simulink model "model"  (R2014a)
(part 5 of 5)

  L_117853438/LConn3 -- T_117853438__/RConn3 -- bus369/LConn1
  T_140066772__/RConn1 -- L_140066772/LConn1
  T_140066772__/RConn2 -- L_140066772/LConn2
  L_140066772/LConn3 -- T_140066772__/RConn3 -- bus370/LConn1
  T_314931464__Csorna_alállomás/RConn1 -- L_314931464/LConn1
  T_314931464__Csorna_alállomás/RConn2 -- L_314931464/LConn2
  L_314931464/LConn3 -- T_314931464__Csorna_alállomás/RConn3 -- bus371/LConn1
  T_313625037__Pápa_alállomás/RConn1 -- L_313625037/LConn1
  T_313625037__Pápa_alállomás/RConn2 -- L_313625037/LConn2
  L_313625037/LConn3 -- T_313625037__Pápa_alállomás/RConn3 -- bus372/LConn1
  T_370667810__/RConn1 -- L_370667810/LConn1
  T_370667810__/RConn2 -- L_370667810/LConn2
  L_370667810/LConn3 -- T_370667810__/RConn3 -- bus373/LConn1
  T_280595113__/RConn1 -- L_280595113/LConn1
  T_280595113__/RConn2 -- L_280595113/LConn2
  L_280595113/LConn3 -- T_280595113__/RConn3 -- bus374/LConn1
  T_294895233__/RConn1 -- L_294895233/LConn1
  T_294895233__/RConn2 -- L_294895233/LConn2
  L_294895233/LConn3 -- T_294895233__/RConn3 -- bus375/LConn1
  T_253119622__Tamási_alállomás/RConn1 -- L_253119622/LConn1
  T_253119622__Tamási_alállomás/RConn2 -- L_253119622/LConn2
  L_253119622/LConn3 -- T_253119622__Tamási_alállomás/RConn3 -- bus376/LConn1
  T_104062255__Sárbogárd_alállomás/RConn1 -- L_104062255/LConn1
  T_104062255__Sárbogárd_alállomás/RConn2 -- L_104062255/LConn2
  L_104062255/LConn3 -- T_104062255__Sárbogárd_alállomás/RConn3 -- bus377/LConn1
  T_135952041_120000_/RConn1 -- L_135952041/LConn1
  T_135952041_120000_/RConn2 -- L_135952041/LConn2
  L_135952041/LConn3 -- T_135952041_120000_/RConn3 -- bus378/LConn1
  T_350948497__/RConn1 -- L_350948497/LConn1
  T_350948497__/RConn2 -- L_350948497/LConn2
  L_350948497/LConn3 -- T_350948497__/RConn3 -- bus379/LConn1
  T_288254104__/RConn1 -- L_288254104/LConn1
  T_288254104__/RConn2 -- L_288254104/LConn2
  L_288254104/LConn3 -- T_288254104__/RConn3 -- bus380/LConn1
  T_234987164__/RConn1 -- L_234987164/LConn1
  T_234987164__/RConn2 -- L_234987164/LConn2
  L_234987164/LConn3 -- T_234987164__/RConn3 -- bus381/LConn1
  T_110253534__/RConn1 -- L_110253534/LConn1
  T_110253534__/RConn2 -- L_110253534/LConn2
  L_110253534/LConn3 -- T_110253534__/RConn3 -- bus382/LConn1
  T_275352278__Kapuvár_alállomás/RConn1 -- L_275352278/LConn1
  T_275352278__Kapuvár_alállomás/RConn2 -- L_275352278/LConn2
  L_275352278/LConn3 -- T_275352278__Kapuvár_alállomás/RConn3 -- bus383/LConn1
  T_287201135__Békés_120_kV_alállomás/RConn1 -- L_287201135/LConn1
  T_287201135__Békés_120_kV_alállomás/RConn2 -- L_287201135/LConn2
  L_287201135/LConn3 -- T_287201135__Békés_120_kV_alállomás/RConn3 -- bus384/LConn1
  T_302147975__Borsodnádasd_alállomás/RConn1 -- L_302147975/LConn1
  T_302147975__Borsodnádasd_alállomás/RConn2 -- L_302147975/LConn2
  L_302147975/LConn3 -- T_302147975__Borsodnádasd_alállomás/RConn3 -- bus385/LConn1
  T_355349327__Öntödei_alállomás/RConn1 -- L_355349327/LConn1
  T_355349327__Öntödei_alállomás/RConn2 -- L_355349327/LConn2
  L_355349327/LConn3 -- T_355349327__Öntödei_alállomás/RConn3 -- bus386/LConn1
  T_103950678__Dunakeszi_alállomás/RConn1 -- L_103950678/LConn1
  T_103950678__Dunakeszi_alállomás/RConn2 -- L_103950678/LConn2
  L_103950678/LConn3 -- T_103950678__Dunakeszi_alállomás/RConn3 -- bus387/LConn1
  T_103950687_120000_Fót_alállomás/RConn1 -- L_103950687/LConn1
  T_103950687_120000_Fót_alállomás/RConn2 -- L_103950687/LConn2
  L_103950687/LConn3 -- T_103950687_120000_Fót_alállomás/RConn3 -- bus388/LConn1
  T_287114424__/RConn1 -- L_287114424/LConn1
  T_287114424__/RConn2 -- L_287114424/LConn2
  L_287114424/LConn3 -- T_287114424__/RConn3 -- bus389/LConn1
  T_291223737__Kunszentmárton_alállomás/RConn1 -- L_291223737/LConn1
  T_291223737__Kunszentmárton_alállomás/RConn2 -- L_291223737/LConn2
  L_291223737/LConn3 -- T_291223737__Kunszentmárton_alállomás/RConn3 -- bus390/LConn1
  T_288736592__Szentes_alállomás/RConn1 -- L_288736592/LConn1
  T_288736592__Szentes_alállomás/RConn2 -- L_288736592/LConn2
  L_288736592/LConn3 -- T_288736592__Szentes_alállomás/RConn3 -- bus391/LConn1
  T_235409083__Sikonda_alállomás/RConn1 -- L_235409083/LConn1
  T_235409083__Sikonda_alállomás/RConn2 -- L_235409083/LConn2
  L_235409083/LConn3 -- T_235409083__Sikonda_alállomás/RConn3 -- bus392/LConn1
  T_331463129__Mindszentgodisa_alállomás/RConn1 -- L_331463129/LConn1
  T_331463129__Mindszentgodisa_alállomás/RConn2 -- L_331463129/LConn2
  L_331463129/LConn3 -- T_331463129__Mindszentgodisa_alállomás/RConn3 -- bus393/LConn1
  T_291442885__Hódmezővásárhely_alállomás/RConn1 -- L_291442885/LConn1
  T_291442885__Hódmezővásárhely_alállomás/RConn2 -- L_291442885/LConn2
  L_291442885/LConn3 -- T_291442885__Hódmezővásárhely_alállomás/RConn3 -- bus394/LConn1
  T_281465215__Nagykőrös_alállomás/RConn1 -- L_281465215/LConn1
  T_281465215__Nagykőrös_alállomás/RConn2 -- L_281465215/LConn2
  L_281465215/LConn3 -- T_281465215__Nagykőrös_alállomás/RConn3 -- bus395/LConn1
  T_153098964__Budaörs_alállomás/RConn1 -- L_153098964/LConn1
  T_153098964__Budaörs_alállomás/RConn2 -- L_153098964/LConn2
  L_153098964/LConn3 -- T_153098964__Budaörs_alállomás/RConn3 -- bus396/LConn1
  T_173251331_120000_Biatorbágy_alállomás/RConn1 -- L_173251331/LConn1
  T_173251331_120000_Biatorbágy_alállomás/RConn2 -- L_173251331/LConn2
  L_173251331/LConn3 -- T_173251331_120000_Biatorbágy_alállomás/RConn3 -- bus397/LConn1
  T_302259884_120000_Szabadbattyán_alállomás/RConn1 -- L_302259884/LConn1
  T_302259884_120000_Szabadbattyán_alállomás/RConn2 -- L_302259884/LConn2
  L_302259884/LConn3 -- T_302259884_120000_Szabadbattyán_alállomás/RConn3 -- bus398/LConn1
  T_214279016__Székesfehérvár_Észak_alállomás/RConn1 -- L_214279016/LConn1
  T_214279016__Székesfehérvár_Észak_alállomás/RConn2 -- L_214279016/LConn2
  L_214279016/LConn3 -- T_214279016__Székesfehérvár_Észak_alállomás/RConn3 -- bus399/LConn1
  T_162874597__Mezőkövesd_alállomás/RConn1 -- L_162874597/LConn1
  T_162874597__Mezőkövesd_alállomás/RConn2 -- L_162874597/LConn2
  L_162874597/LConn3 -- T_162874597__Mezőkövesd_alállomás/RConn3 -- bus400/LConn1
  T_235599317__Füzesabony_alállomás/RConn1 -- L_235599317/LConn1
  T_235599317__Füzesabony_alállomás/RConn2 -- L_235599317/LConn2
  L_235599317/LConn3 -- T_235599317__Füzesabony_alállomás/RConn3 -- bus401/LConn1
  T_271034091__Baja_Dunapart_alállomás/RConn1 -- L_271034091/LConn1
  T_271034091__Baja_Dunapart_alállomás/RConn2 -- L_271034091/LConn2
  L_271034091/LConn3 -- T_271034091__Baja_Dunapart_alállomás/RConn3 -- bus402/LConn1
  T_283715413__Baja_120_kV_alállomás/RConn1 -- L_283715413/LConn1
  T_283715413__Baja_120_kV_alállomás/RConn2 -- L_283715413/LConn2
  L_283715413/LConn3 -- T_283715413__Baja_120_kV_alállomás/RConn3 -- bus403/LConn1
  T_288863210__/RConn1 -- L_288863210/LConn1
  T_288863210__/RConn2 -- L_288863210/LConn2
  L_288863210/LConn3 -- T_288863210__/RConn3 -- bus404/LConn1
  T_312136451__/RConn1 -- L_312136451/LConn1
  T_312136451__/RConn2 -- L_312136451/LConn2
  L_312136451/LConn3 -- T_312136451__/RConn3 -- bus405/LConn1
  T_307229690__/RConn1 -- L_307229690/LConn1
  T_307229690__/RConn2 -- L_307229690/LConn2
  L_307229690/LConn3 -- T_307229690__/RConn3 -- bus406/LConn1
  T_128526607__Eger_Észak_alállomás/RConn1 -- L_128526607/LConn1
  T_128526607__Eger_Észak_alállomás/RConn2 -- L_128526607/LConn2
  L_128526607/LConn3 -- T_128526607__Eger_Észak_alállomás/RConn3 -- bus407/LConn1
  T_294585306__/RConn1 -- L_294585306/LConn1
  T_294585306__/RConn2 -- L_294585306/LConn2
  L_294585306/LConn3 -- T_294585306__/RConn3 -- bus408/LConn1
  T_294690169__Hejőcsaba_alállomás/RConn1 -- L_294690169/LConn1
  T_294690169__Hejőcsaba_alállomás/RConn2 -- L_294690169/LConn2
  L_294690169/LConn3 -- T_294690169__Hejőcsaba_alállomás/RConn3 -- bus409/LConn1
  T_121135019_120000;20000_120_20_kV_s_Barcsi_tarnszformátor_állomás/RConn1 -- L_121135019/LConn1
  T_121135019_120000;20000_120_20_kV_s_Barcsi_tarnszformátor_állomás/RConn2 -- L_121135019/LConn2
  L_121135019/LConn3 -- T_121135019_120000;20000_120_20_kV_s_Barcsi_tarnszformátor_állomás/RConn3 -- bus410/LConn1
  T_104062252__/RConn1 -- L_104062252/LConn1
  T_104062252__/RConn2 -- L_104062252/LConn2
  L_104062252/LConn3 -- T_104062252__/RConn3 -- bus411/LConn1
  T_283021123__Szabadszállás_alállomás/RConn1 -- L_283021123/LConn1
  T_283021123__Szabadszállás_alállomás/RConn2 -- L_283021123/LConn2
  L_283021123/LConn3 -- T_283021123__Szabadszállás_alállomás/RConn3 -- bus412/LConn1
  T_254603237_120000;10000_Népliget/RConn1 -- L_254603237/LConn1
  T_254603237_120000;10000_Népliget/RConn2 -- L_254603237/LConn2
  L_254603237/LConn3 -- T_254603237_120000;10000_Népliget/RConn3 -- bus413/LConn1
  T_288721741__Dunaújváros_II__132_22_kV_os_transzformátor_állomás/RConn1 -- L_288721741/LConn1
  T_288721741__Dunaújváros_II__132_22_kV_os_transzformátor_állomás/RConn2 -- L_288721741/LConn2
  L_288721741/LConn3 -- T_288721741__Dunaújváros_II__132_22_kV_os_transzformátor_állomás/RConn3 -- bus414/LConn1
  T_243726196_120000;11000_Kanizsavár_alállomás/RConn1 -- L_243726196/LConn1
  T_243726196_120000;11000_Kanizsavár_alállomás/RConn2 -- L_243726196/LConn2
  L_243726196/LConn3 -- T_243726196_120000;11000_Kanizsavár_alállomás/RConn3 -- bus415/LConn1
  T_283273093__Csongrád_alállomás/RConn1 -- L_283273093/LConn1
  T_283273093__Csongrád_alállomás/RConn2 -- L_283273093/LConn2
  L_283273093/LConn3 -- T_283273093__Csongrád_alállomás/RConn3 -- bus416/LConn1
  T_103984593__/RConn1 -- L_103984593/LConn1
  T_103984593__/RConn2 -- L_103984593/LConn2
  L_103984593/LConn3 -- T_103984593__/RConn3 -- bus417/LConn1
  T_289912791__/RConn1 -- L_289912791/LConn1
  T_289912791__/RConn2 -- L_289912791/LConn2
  L_289912791/LConn3 -- T_289912791__/RConn3 -- bus418/LConn1
  T_299521957__Salgótarján,_Művésztelepi_alállomás/RConn1 -- L_299521957/LConn1
  T_299521957__Salgótarján,_Művésztelepi_alállomás/RConn2 -- L_299521957/LConn2
  L_299521957/LConn3 -- T_299521957__Salgótarján,_Művésztelepi_alállomás/RConn3 -- bus419/LConn1
  T_215137750_120000_Rákosfalva_alállomás/RConn1 -- L_215137750/LConn1
  T_215137750_120000_Rákosfalva_alállomás/RConn2 -- L_215137750/LConn2
  L_215137750/LConn3 -- T_215137750_120000_Rákosfalva_alállomás/RConn3 -- bus420/LConn1
  T_281860578__Károlyfalva_alállomás/RConn1 -- L_281860578/LConn1
  T_281860578__Károlyfalva_alállomás/RConn2 -- L_281860578/LConn2
  L_281860578/LConn3 -- T_281860578__Károlyfalva_alállomás/RConn3 -- bus421/LConn1
  T_304280556__/RConn1 -- L_304280556/LConn1
  T_304280556__/RConn2 -- L_304280556/LConn2
  L_304280556/LConn3 -- T_304280556__/RConn3 -- bus422/LConn1
  T_172048867__ELMŰ_Rózsakert_132_10_kV_alállomás/RConn1 -- L_172048867/LConn1
  T_172048867__ELMŰ_Rózsakert_132_10_kV_alállomás/RConn2 -- L_172048867/LConn2
  L_172048867/LConn3 -- T_172048867__ELMŰ_Rózsakert_132_10_kV_alállomás/RConn3 -- bus423/LConn1
  T_172049204__Diósd_alállomás/RConn1 -- L_172049204/LConn1
  T_172049204__Diósd_alállomás/RConn2 -- L_172049204/LConn2
  L_172049204/LConn3 -- T_172049204__Diósd_alállomás/RConn3 -- bus424/LConn1
  T_100848980__Érd/RConn1 -- L_100848980/LConn1
  T_100848980__Érd/RConn2 -- L_100848980/LConn2
  L_100848980/LConn3 -- T_100848980__Érd/RConn3 -- bus425/LConn1
  T_285581278__/RConn1 -- L_285581278/LConn1
  T_285581278__/RConn2 -- L_285581278/LConn2
  L_285581278/LConn3 -- T_285581278__/RConn3 -- bus426/LConn1
  T_244038276_220000;120000_Oroszlány_alállomás/RConn1 -- L_244038276/LConn1
  T_244038276_220000;120000_Oroszlány_alállomás/RConn2 -- L_244038276/LConn2
  L_244038276/LConn3 -- T_244038276_220000;120000_Oroszlány_alállomás/RConn3 -- bus427/LConn1
  T_354667530__/RConn1 -- L_354667530/LConn1
  T_354667530__/RConn2 -- L_354667530/LConn2
  L_354667530/LConn3 -- T_354667530__/RConn3 -- bus428/LConn1
  T_195155625__/RConn1 -- L_195155625/LConn1
  T_195155625__/RConn2 -- L_195155625/LConn2
  L_195155625/LConn3 -- T_195155625__/RConn3 -- bus429/LConn1
  T_142106943_400000_Gönyü_400kV_alállomás/RConn1 -- L_142106943/LConn1
  T_142106943_400000_Gönyü_400kV_alállomás/RConn2 -- L_142106943/LConn2
  L_142106943/LConn3 -- T_142106943_400000_Gönyü_400kV_alállomás/RConn3 -- bus430/LConn1
  T_142109093__Albertirsa_alállomás/RConn1 -- L_142109093/LConn1
  T_142109093__Albertirsa_alállomás/RConn2 -- L_142109093/LConn2
  L_142109093/LConn3 -- T_142109093__Albertirsa_alállomás/RConn3 -- bus431/LConn1
  T_203815422_400000;220000;110000;35000_Мукачеве_400/RConn1 -- L_203815422/LConn1
  T_203815422_400000;220000;110000;35000_Мукачеве_400/RConn2 -- L_203815422/LConn2
  L_203815422/LConn3 -- T_203815422_400000;220000;110000;35000_Мукачеве_400/RConn3 -- bus432/LConn1
  T_101158766__/RConn1 -- L_101158766/LConn1
  T_101158766__/RConn2 -- L_101158766/LConn2
  L_101158766/LConn3 -- T_101158766__/RConn3 -- bus433/LConn1
  T_89109496__/RConn1 -- L_89109496/LConn1
  T_89109496__/RConn2 -- L_89109496/LConn2
  L_89109496/LConn3 -- T_89109496__/RConn3 -- bus434/LConn1
